simulink library "CTRL_LO_ST3"  (R2023b)
settings: Solver=VariableStepAuto  StartTime=0.0  StopTime=10.0  RelTol=1e-3
undefined symbols (not defined in the file or in its folder): CTRL_LO_p_TqMotLoLim_Nm, CTRL_LO_p_TqMotUpLim_Nm, CTRL_LO_ST3_p_SwtTqFrReRat_na, CTRL_LO_ST3_p_SwtTqYawFrReRat_na, CTRL_LO_ST3_p_TqFrReRat1_na, CTRL_LO_ST3_p_TqFrReRat2_na, CTRL_LO_ST3_p_TqFrReRat3_na, CTRL_LO_ST3_p_TqYawFrReRat1_na, CTRL_LO_ST3_p_TqYawFrReRat2_na, CTRL_LO_ST3_p_TqYawFrReRat3_na, p_RadWhlDynFr_m, p_RadWhlDynRe_m, p_RatGearFr_na, p_trackFr_m, p_trackRe_m
libraries: simulink x1
settings Model: Creator=blatak  LastModifiedBy=blatak

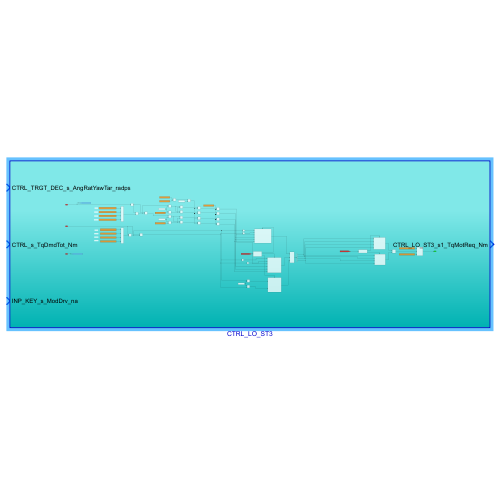
[thumbnail: Simulink's stored preview of the top-level diagram]
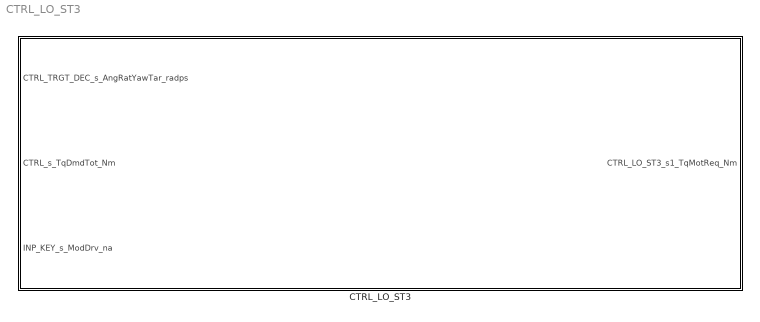
== system CTRL_LO_ST3 ==
  CTRL_LO_ST3 : Subsystem

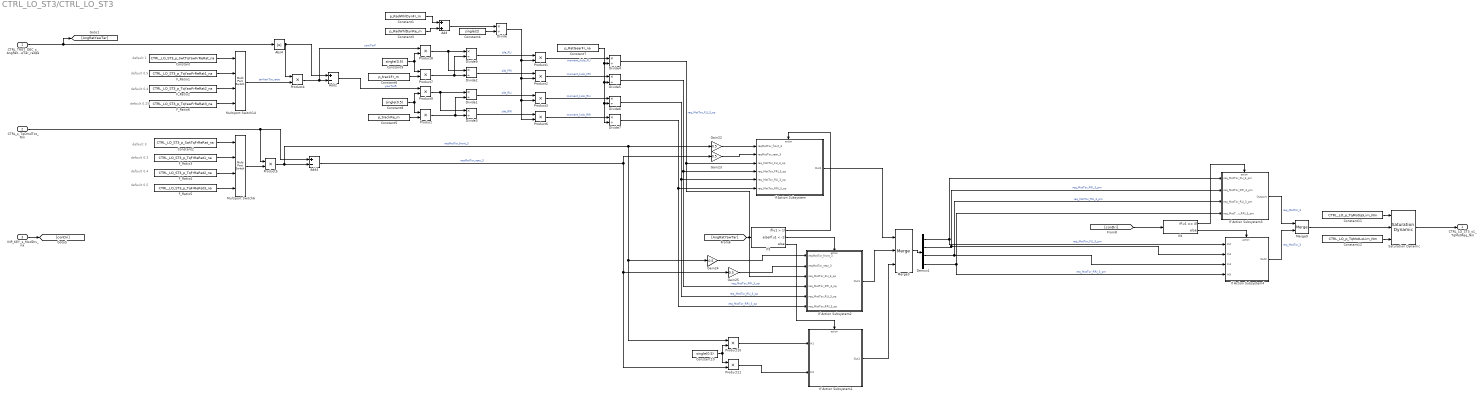
== system CTRL_LO_ST3/CTRL_LO_ST3 ==
  note: default 1
  note: default 0.5
  note: default 0.4
  note: default 0.25
  note: default 0.4
  note: default 0.5
  note: default 3
  note: default 0.3
  CTRL_TRGT_DEC_s_AngRatYawTar_radps : Inport
  CTRL_s_TqDmdTot_Nm : Inport  Port=2
  INP_KEY_s_ModDrv_na : Inport  Port=3
  Abs4 : Abs  SaturateOnIntegerOverflow=off
  Add : Sum
  Add2 : Sum  Inputs=+-
  Add4 : Sum  Inputs=+-
  Constant : Constant  Value=CTRL_LO_ST3_p_SwtTqYawFrReRat_na
  Constant1 : Constant  Value=p_RadWhlDynFr_m
  Constant10 : Constant  Value=single(0.5)
  Constant11 : Constant  Value=CTRL_LO_p_TqMotUpLim_Nm
  Constant12 : Constant  Value=CTRL_LO_p_TqMotLoLim_Nm
  Constant2 : Constant  Value=CTRL_LO_ST3_p_SwtTqFrReRat_na
  Constant3 : Constant  Value=p_RadWhlDynRe_m
  Constant4 : Constant  Value=single(2)
  Constant5 : Constant  Value=p_trackRe_m
  Constant6 : Constant  Value=p_trackFr_m
  Constant7 : Constant  Value=p_RatGearFr_na
  Constant8 : Constant  Value=single(0.5)
  Constant9 : Constant  Value=single(0.5)
  Demux1 : Demux
  Divide{,1..7,9} (9 alike) : Product  Inputs=*/
  F_Ratio1 : Constant  Value=CTRL_LO_ST3_p_TqYawFrReRat1_na
  F_Ratio2 : Constant  Value=CTRL_LO_ST3_p_TqYawFrReRat2_na
  F_Ratio3 : Constant  Value=CTRL_LO_ST3_p_TqFrReRat1_na
  F_Ratio4 : Constant  Value=CTRL_LO_ST3_p_TqFrReRat2_na
  F_Ratio5 : Constant  Value=CTRL_LO_ST3_p_TqFrReRat3_na
  F_Ratio6 : Constant  Value=CTRL_LO_ST3_p_TqYawFrReRat3_na
  Gain{22..25} (4 alike) : Gain  Gain=0.5
  If Action Subsystem : Subsystem  TreatAsAtomicUnit=on
  If Action Subsystem1 : Subsystem  TreatAsAtomicUnit=on
  If Action Subsystem2 : Subsystem  TreatAsAtomicUnit=on
  If Action Subsystem3 : Subsystem  TreatAsAtomicUnit=on
  If Action Subsystem4 : Subsystem  TreatAsAtomicUnit=on
  If3 : If  IfExpression=u1 > 1  ElseIfExpressions=u1 < -1
  If4 : If  IfExpression=u1 == 4
  Merge3 : Merge  Inputs=3
  Merge9 : Merge
  Multiport Switch14 : MultiPortSwitch  SaturateOnIntegerOverflow=off  InputSameDT=off
  Multiport Switch6 : MultiPortSwitch  SaturateOnIntegerOverflow=off  InputSameDT=off
  Product{,1..11} (12 alike) : Product
  Saturation Dynamic : simulink/Discontinuities/Saturation Dynamic  OutMin=[]  OutMax=[]  OutDataTypeStr=Inherit: Same as second input  OutDataType=fixdt(1, 16)  OutScaling=2^-10  DoSatur=off
  CTRL_LO_ST3_s1_TqMotReq_Nm : Outport
  wires:
  If3/2 -> If Action Subsystem2/Action
  Demux1/2 -> If Action Subsystem4/2(In3), If Action Subsystem3/2(req_MotTor_FRI_3_pm)  "req_MotTor_FRI_3_pm"
  If3/1 -> If Action Subsystem/Action
  Product5/1 -> Product10/1, Gain24/1, Gain22/1, Add4/2  "reqMotTor_front_3"
  CTRL_TRGT_DEC_s_AngRatYawTar_radps/1 -> [AngRatYawTar], Abs4/1
  Demux1/3 -> If Action Subsystem4/3(In4), If Action Subsystem3/3(req_MotTor_RLI_3_pm)  "req_MotTor_RLI_3_pm"
  If Action Subsystem/1(Out1) -> Merge3/1
  Demux1/1 -> If Action Subsystem4/1(In2), If Action Subsystem3/1(req_MotTor_FLI_3_pm)  "req_MotTor_FLI_3_pm"
  Divide5/1 -> If Action Subsystem2/4(req_MotTor_FRI_3_op), If Action Subsystem/4(req_MotTor_FRI_3_op)  "req_MotTor_FRI_3_op"
  Product4/1 -> Product8/1, Add2/2  "yawTorF"
  F_Ratio1/1 -> Multiport Switch14/2
  F_Ratio6/1 -> Multiport Switch14/4
  Gain23/1 -> If Action Subsystem/2(reqMotTor_rear_3)
  Divide6/1 -> If Action Subsystem2/5(req_MotTor_RLI_3_op), If Action Subsystem/5(req_MotTor_RLI_3_op)  "req_MotTor_RLI_3_op"
  Add2/1 -> Product9/1  "yawTorR"
  If4/2 -> If Action Subsystem4/Action
  If Action Subsystem4/1(Out2) -> Merge9/2  "req_MotTor_3"
  F_Ratio2/1 -> Multiport Switch14/3
  CTRL_s_TqDmdTot_Nm/1 -> Add4/1, Product5/1
  Abs4/1 -> Add2/1, Product4/1
  Multiport Switch14/1 -> Product4/2  "tarYawTor_ratio"
  Constant2/1 -> Multiport Switch6/1
  F_Ratio3/1 -> Multiport Switch6/2
  Divide4/1 -> If Action Subsystem2/3(req_MotTor_FLI_3_op), If Action Subsystem/3(req_MotTor_FLI_3_op)  "req_MotTor_FLI_3_op"
  Product11/1 -> If Action Subsystem1/2(In2)
  F_Ratio5/1 -> Multiport Switch6/4
  Multiport Switch6/1 -> Product5/2
  Product10/1 -> If Action Subsystem1/1(In1)
  If4/1 -> If Action Subsystem3/Action
  If Action Subsystem2/1(Out1) -> Merge3/2
  F_Ratio4/1 -> Multiport Switch6/3
  [AngRatYawTar] -> If3/1
  If Action Subsystem3/1(Outport) -> Merge9/1  "req_MotTor_3"
  If3/3 -> If Action Subsystem1/Action
  Divide7/1 -> If Action Subsystem2/6(req_MotTor_RRI_3_op), If Action Subsystem/6(req_MotTor_RRI_3_op)  "req_MotTor_RRI_3_op"
  Merge3/1 -> Demux1/1
  Add4/1 -> Product11/2, Gain25/1, Gain23/1  "reqMotTor_rear_3"
  Gain22/1 -> If Action Subsystem/1(reqMotTor_front_3)
  [conDri] -> If4/1
  Gain25/1 -> If Action Subsystem2/2(reqMotTor_rear_3)
  Gain24/1 -> If Action Subsystem2/1(reqMotTor_front_3)
  Constant/1 -> Multiport Switch14/1
  Demux1/4 -> If Action Subsystem3/4(req_MotTor_RRI_3_pm), If Action Subsystem4/4(In5)  "req_MotTor_RRI_3_pm"
  If Action Subsystem1/1(Out1) -> Merge3/3
  Constant6/1 -> Product7/2
  Product2/1 -> Divide5/1  "moment_kolo_FRI"
  Product7/1 -> Divide2/2, Divide9/2
  Product1/1 -> Divide4/1  "moment_kolo_FLI"
  Divide/1 -> Product6/2, Product3/2, Product2/2, Product1/2
  Product/1 -> Divide3/2, Divide1/2
  Divide3/1 -> Product6/1  "sila_RRI"
  Constant5/1 -> Product/2
  Divide1/1 -> Product3/1  "sila_RLI"
  Product6/1 -> Divide7/1  "moment_kolo_RRI"
  Divide9/1 -> Product1/1  "sila_FLI"
  Product8/1 -> Divide9/1, Divide2/1
  Constant7/1 -> Divide4/2, Divide7/2, Divide6/2, Divide5/2
  Divide2/1 -> Product2/1  "sila_FRI"
  Product3/1 -> Divide6/1  "moment_kolo_RLI"
  Product9/1 -> Divide1/1, Divide3/1
  Constant4/1 -> Divide/2
  Add/1 -> Divide/1
  Constant1/1 -> Add/1
  Constant3/1 -> Add/2
  Constant8/1 -> Product9/2, Product/1
  Constant9/1 -> Product7/1, Product8/2
  INP_KEY_s_ModDrv_na/1 -> [conDri]
  Constant10/1 -> Product11/1, Product10/2
  Merge9/1 -> Saturation Dynamic/2
  Constant12/1 -> Saturation Dynamic/3
  Constant11/1 -> Saturation Dynamic/1
  Saturation Dynamic/1 -> CTRL_LO_ST3_s1_TqMotReq_Nm/1

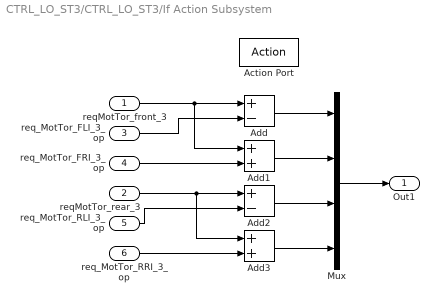
== system CTRL_LO_ST3/CTRL_LO_ST3/If Action Subsystem ==
  reqMotTor_front_3 : Inport
  reqMotTor_rear_3 : Inport  Port=2
  req_MotTor_FLI_3_op : Inport  Port=3
  req_MotTor_FRI_3_op : Inport  Port=4
  req_MotTor_RLI_3_op : Inport  Port=5
  req_MotTor_RRI_3_op : Inport  Port=6
  Action Port : ActionPort  ActionPortLabel=if(u1 > 1)
  Add : Sum  Inputs=+-
  Add1 : Sum
  Add2 : Sum  Inputs=+-
  Add3 : Sum
  Mux : Mux
  Out1 : Outport
  wires:
  req_MotTor_FRI_3_op/1 -> Add1/2
  reqMotTor_front_3/1 -> Add1/1, Add/1
  Add1/1 -> Mux/2
  Add2/1 -> Mux/3
  req_MotTor_RRI_3_op/1 -> Add3/2
  reqMotTor_rear_3/1 -> Add3/1, Add2/1
  Mux/1 -> Out1/1
  req_MotTor_FLI_3_op/1 -> Add/2
  Add3/1 -> Mux/4
  req_MotTor_RLI_3_op/1 -> Add2/2
  Add/1 -> Mux/1

== system CTRL_LO_ST3/CTRL_LO_ST3/If Action Subsystem1 ==
  In1 : Inport
  In2 : Inport  Port=2
  Action Port : ActionPort  ActionPortLabel=else
  Mux : Mux
  Out1 : Outport
  wires:
  In2/1 -> Mux/4, Mux/3
  In1/1 -> Mux/2, Mux/1
  Mux/1 -> Out1/1

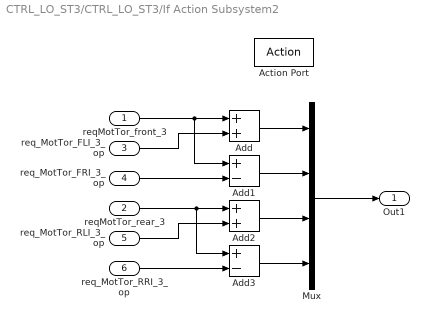
== system CTRL_LO_ST3/CTRL_LO_ST3/If Action Subsystem2 ==
  reqMotTor_front_3 : Inport
  reqMotTor_rear_3 : Inport  Port=2
  req_MotTor_FLI_3_op : Inport  Port=3
  req_MotTor_FRI_3_op : Inport  Port=4
  req_MotTor_RLI_3_op : Inport  Port=5
  req_MotTor_RRI_3_op : Inport  Port=6
  Action Port : ActionPort  ActionPortLabel=elseif(u1 < -1)
  Add : Sum
  Add1 : Sum  Inputs=+-
  Add2 : Sum
  Add3 : Sum  Inputs=+-
  Mux : Mux
  Out1 : Outport
  wires:
  reqMotTor_rear_3/1 -> Add3/1, Add2/1
  req_MotTor_RLI_3_op/1 -> Add2/2
  Mux/1 -> Out1/1
  Add/1 -> Mux/1
  req_MotTor_RRI_3_op/1 -> Add3/2
  req_MotTor_FLI_3_op/1 -> Add/2
  Add2/1 -> Mux/3
  reqMotTor_front_3/1 -> Add1/1, Add/1
  Add1/1 -> Mux/2
  Add3/1 -> Mux/4
  req_MotTor_FRI_3_op/1 -> Add1/2

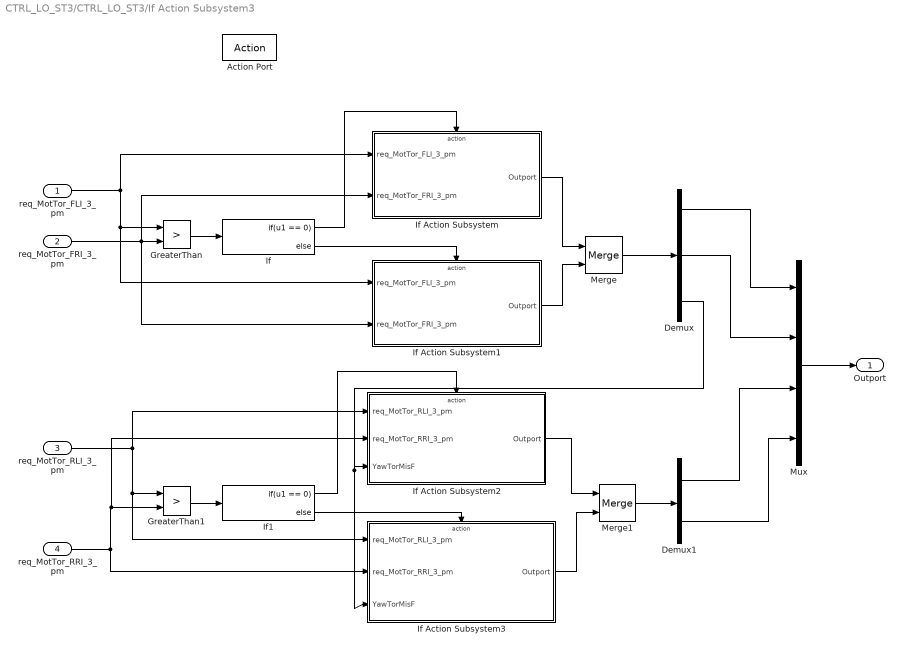
== system CTRL_LO_ST3/CTRL_LO_ST3/If Action Subsystem3 ==
  req_MotTor_FLI_3_pm : Inport
  req_MotTor_FRI_3_pm : Inport  Port=2
  req_MotTor_RLI_3_pm : Inport  Port=3
  req_MotTor_RRI_3_pm : Inport  Port=4
  Action Port : ActionPort  ActionPortLabel=if(u1 == 4)
  Demux : Demux  Outputs=3
  Demux1 : Demux  Outputs=2
  GreaterThan : RelationalOperator  Operator=>  OutDataTypeStr=boolean  RndMeth=Simplest  InputSameDT=off
  GreaterThan1 : RelationalOperator  Operator=>  OutDataTypeStr=boolean  RndMeth=Simplest  InputSameDT=off
  If : If  IfExpression=u1 == 0
  If Action Subsystem : Subsystem  TreatAsAtomicUnit=on
  If Action Subsystem1 : Subsystem  TreatAsAtomicUnit=on
  If Action Subsystem2 : Subsystem  TreatAsAtomicUnit=on
  If Action Subsystem3 : Subsystem  TreatAsAtomicUnit=on
  If1 : If  IfExpression=u1 == 0
  Merge : Merge
  Merge1 : Merge
  Mux : Mux
  Outport : Outport
  wires:
  GreaterThan/1 -> If/1
  If/1 -> If Action Subsystem/Action
  If1/1 -> If Action Subsystem2/Action
  If1/2 -> If Action Subsystem3/Action
  GreaterThan1/1 -> If1/1
  req_MotTor_RLI_3_pm/1 -> If Action Subsystem2/1(req_MotTor_RLI_3_pm), If Action Subsystem3/1(req_MotTor_RLI_3_pm), GreaterThan1/1
  req_MotTor_FRI_3_pm/1 -> If Action Subsystem1/2(req_MotTor_FRI_3_pm), If Action Subsystem/2(req_MotTor_FRI_3_pm), GreaterThan/2
  req_MotTor_RRI_3_pm/1 -> If Action Subsystem3/2(req_MotTor_RRI_3_pm), If Action Subsystem2/2(req_MotTor_RRI_3_pm), GreaterThan1/2
  If/2 -> If Action Subsystem1/Action
  req_MotTor_FLI_3_pm/1 -> If Action Subsystem/1(req_MotTor_FLI_3_pm), If Action Subsystem1/1(req_MotTor_FLI_3_pm), GreaterThan/1
  If Action Subsystem/1(Outport) -> Merge/1
  If Action Subsystem1/1(Outport) -> Merge/2
  If Action Subsystem2/1(Outport) -> Merge1/1
  If Action Subsystem3/1(Outport) -> Merge1/2
  Merge/1 -> Demux/1
  Demux/3 -> If Action Subsystem3/3(YawTorMisF), If Action Subsystem2/3(YawTorMisF)
  Merge1/1 -> Demux1/1
  Demux/1 -> Mux/1
  Demux/2 -> Mux/2
  Demux1/1 -> Mux/3
  Demux1/2 -> Mux/4
  Mux/1 -> Outport/1

== system CTRL_LO_ST3/CTRL_LO_ST3/If Action Subsystem4 ==
  In2 : Inport
  In3 : Inport  Port=2
  In4 : Inport  Port=3
  In5 : Inport  Port=4
  Action Port : ActionPort  ActionPortLabel=else
  Mux : Mux
  Out2 : Outport
  wires:
  Mux/1 -> Out2/1
  In5/1 -> Mux/4
  In3/1 -> Mux/2
  In4/1 -> Mux/3
  In2/1 -> Mux/1

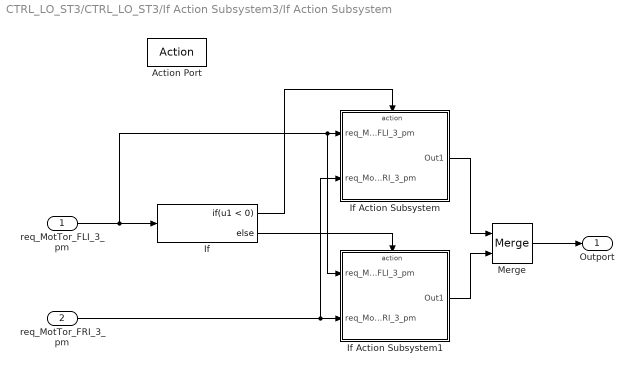
== system CTRL_LO_ST3/CTRL_LO_ST3/If Action Subsystem3/If Action Subsystem ==
  req_MotTor_FLI_3_pm : Inport
  req_MotTor_FRI_3_pm : Inport  Port=2
  Action Port : ActionPort  ActionPortLabel=if(u1 == 0)
  If : If  IfExpression=u1 < 0
  If Action Subsystem : Subsystem  TreatAsAtomicUnit=on
  If Action Subsystem1 : Subsystem  TreatAsAtomicUnit=on
  Merge : Merge
  Outport : Outport
  wires:
  If/1 -> If Action Subsystem/Action
  If/2 -> If Action Subsystem1/Action
  req_MotTor_FRI_3_pm/1 -> If Action Subsystem1/2(req_MotTor_FRI_3_pm), If Action Subsystem/2(req_MotTor_FRI_3_pm)
  req_MotTor_FLI_3_pm/1 -> If Action Subsystem1/1(req_MotTor_FLI_3_pm), If Action Subsystem/1(req_MotTor_FLI_3_pm), If/1
  If Action Subsystem/1(Out1) -> Merge/1
  If Action Subsystem1/1(Out1) -> Merge/2
  Merge/1 -> Outport/1

== system CTRL_LO_ST3/CTRL_LO_ST3/If Action Subsystem3/If Action Subsystem1 ==
  req_MotTor_FLI_3_pm : Inport
  req_MotTor_FRI_3_pm : Inport  Port=2
  Action Port : ActionPort  ActionPortLabel=else
  If : If  IfExpression=u1 < 0
  If Action Subsystem : Subsystem  TreatAsAtomicUnit=on
  If Action Subsystem1 : Subsystem  TreatAsAtomicUnit=on
  Merge : Merge
  Outport : Outport
  wires:
  If/1 -> If Action Subsystem/Action
  If/2 -> If Action Subsystem1/Action
  req_MotTor_FRI_3_pm/1 -> If Action Subsystem1/2(req_MotTor_FRI_3_pm), If Action Subsystem/2(req_MotTor_FRI_3_pm), If/1
  req_MotTor_FLI_3_pm/1 -> If Action Subsystem1/1(req_MotTor_FLI_3_pm), If Action Subsystem/1(req_MotTor_FLI_3_pm)
  If Action Subsystem/1(Out1) -> Merge/1
  If Action Subsystem1/1(Out1) -> Merge/2
  Merge/1 -> Outport/1

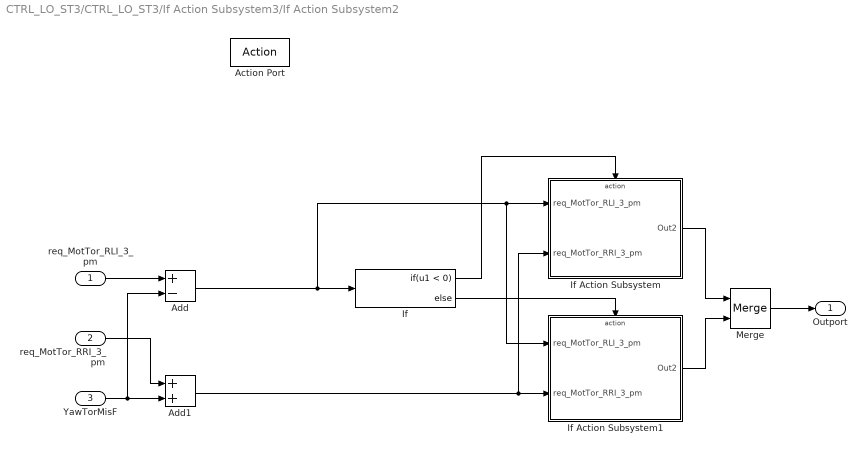
== system CTRL_LO_ST3/CTRL_LO_ST3/If Action Subsystem3/If Action Subsystem2 ==
  req_MotTor_RLI_3_pm : Inport
  req_MotTor_RRI_3_pm : Inport  Port=2
  YawTorMisF : Inport  Port=3
  Action Port : ActionPort  ActionPortLabel=if(u1 == 0)
  Add : Sum  Inputs=+-
  Add1 : Sum
  If : If  IfExpression=u1 < 0
  If Action Subsystem : Subsystem  TreatAsAtomicUnit=on
  If Action Subsystem1 : Subsystem  TreatAsAtomicUnit=on
  Merge : Merge
  Outport : Outport
  wires:
  Add/1 -> If/1, If Action Subsystem1/1(req_MotTor_RLI_3_pm), If Action Subsystem/1(req_MotTor_RLI_3_pm)
  If/1 -> If Action Subsystem/Action
  Add1/1 -> If Action Subsystem1/2(req_MotTor_RRI_3_pm), If Action Subsystem/2(req_MotTor_RRI_3_pm)
  If/2 -> If Action Subsystem1/Action
  req_MotTor_RRI_3_pm/1 -> Add1/1
  req_MotTor_RLI_3_pm/1 -> Add/1
  YawTorMisF/1 -> Add1/2, Add/2
  If Action Subsystem/1(Out2) -> Merge/1
  If Action Subsystem1/1(Out2) -> Merge/2
  Merge/1 -> Outport/1

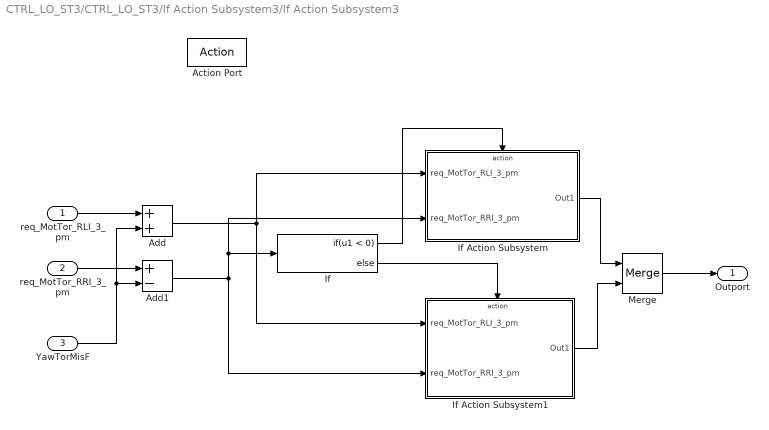
== system CTRL_LO_ST3/CTRL_LO_ST3/If Action Subsystem3/If Action Subsystem3 ==
  req_MotTor_RLI_3_pm : Inport
  req_MotTor_RRI_3_pm : Inport  Port=2
  YawTorMisF : Inport  Port=3
  Action Port : ActionPort  ActionPortLabel=else
  Add : Sum
  Add1 : Sum  Inputs=+-
  If : If  IfExpression=u1 < 0
  If Action Subsystem : Subsystem  TreatAsAtomicUnit=on
  If Action Subsystem1 : Subsystem  TreatAsAtomicUnit=on
  Merge : Merge
  Outport : Outport
  wires:
  req_MotTor_RLI_3_pm/1 -> Add/1
  Add/1 -> If Action Subsystem1/1(req_MotTor_RLI_3_pm), If Action Subsystem/1(req_MotTor_RLI_3_pm)
  req_MotTor_RRI_3_pm/1 -> Add1/1
  If/2 -> If Action Subsystem1/Action
  Add1/1 -> If Action Subsystem1/2(req_MotTor_RRI_3_pm), If Action Subsystem/2(req_MotTor_RRI_3_pm), If/1
  If/1 -> If Action Subsystem/Action
  YawTorMisF/1 -> Add/2, Add1/2
  If Action Subsystem/1(Out1) -> Merge/1
  If Action Subsystem1/1(Out1) -> Merge/2
  Merge/1 -> Outport/1

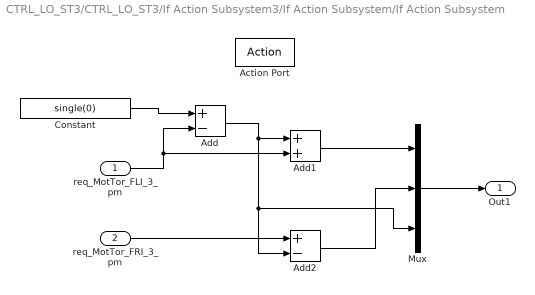
== system CTRL_LO_ST3/CTRL_LO_ST3/If Action Subsystem3/If Action Subsystem/If Action Subsystem ==
  req_MotTor_FLI_3_pm : Inport
  req_MotTor_FRI_3_pm : Inport  Port=2
  Action Port : ActionPort  ActionPortLabel=if(u1 < 0)
  Add : Sum  Inputs=+-
  Add1 : Sum
  Add2 : Sum  Inputs=+-
  Constant : Constant  Value=single(0)
  Mux : Mux  Inputs=3
  Out1 : Outport
  wires:
  Add1/1 -> Mux/1
  Add/1 -> Add2/2, Mux/3, Add1/1
  Add2/1 -> Mux/2
  Constant/1 -> Add/1
  Mux/1 -> Out1/1
  req_MotTor_FRI_3_pm/1 -> Add2/1
  req_MotTor_FLI_3_pm/1 -> Add1/2, Add/2

== system CTRL_LO_ST3/CTRL_LO_ST3/If Action Subsystem3/If Action Subsystem/If Action Subsystem1 ==
  req_MotTor_FLI_3_pm : Inport
  req_MotTor_FRI_3_pm : Inport  Port=2
  Action Port : ActionPort  ActionPortLabel=else
  Constant : Constant  Value=single(0)
  Mux : Mux  Inputs=3
  Out1 : Outport
  wires:
  Mux/1 -> Out1/1
  req_MotTor_FRI_3_pm/1 -> Mux/2
  req_MotTor_FLI_3_pm/1 -> Mux/1
  Constant/1 -> Mux/3

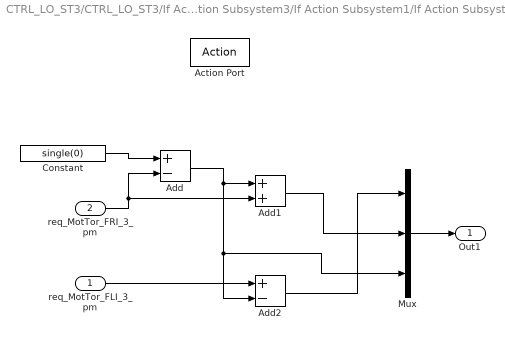
== system CTRL_LO_ST3/CTRL_LO_ST3/If Action Subsystem3/If Action Subsystem1/If Action Subsystem ==
  req_MotTor_FLI_3_pm : Inport
  req_MotTor_FRI_3_pm : Inport  Port=2
  Action Port : ActionPort  ActionPortLabel=if(u1 < 0)
  Add : Sum  Inputs=+-
  Add1 : Sum
  Add2 : Sum  Inputs=+-
  Constant : Constant  Value=single(0)
  Mux : Mux  Inputs=3
  Out1 : Outport
  wires:
  req_MotTor_FLI_3_pm/1 -> Add2/1
  Add/1 -> Add2/2, Mux/3, Add1/1
  Mux/1 -> Out1/1
  Add2/1 -> Mux/1
  Add1/1 -> Mux/2
  req_MotTor_FRI_3_pm/1 -> Add1/2, Add/2
  Constant/1 -> Add/1

== system CTRL_LO_ST3/CTRL_LO_ST3/If Action Subsystem3/If Action Subsystem1/If Action Subsystem1 ==
  req_MotTor_FLI_3_pm : Inport
  req_MotTor_FRI_3_pm : Inport  Port=2
  Action Port : ActionPort  ActionPortLabel=else
  Constant : Constant  Value=single(0)
  Mux : Mux  Inputs=3
  Out1 : Outport
  wires:
  Mux/1 -> Out1/1
  req_MotTor_FLI_3_pm/1 -> Mux/1
  Constant/1 -> Mux/3
  req_MotTor_FRI_3_pm/1 -> Mux/2

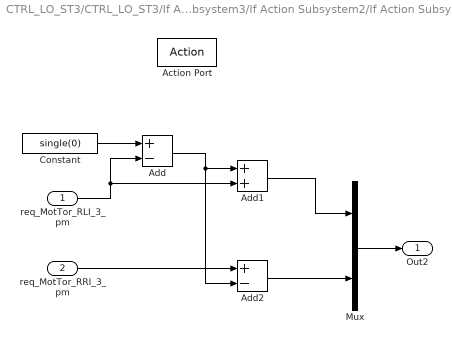
== system CTRL_LO_ST3/CTRL_LO_ST3/If Action Subsystem3/If Action Subsystem2/If Action Subsystem ==
  req_MotTor_RLI_3_pm : Inport
  req_MotTor_RRI_3_pm : Inport  Port=2
  Action Port : ActionPort  ActionPortLabel=if(u1 < 0)
  Add : Sum  Inputs=+-
  Add1 : Sum
  Add2 : Sum  Inputs=+-
  Constant : Constant  Value=single(0)
  Mux : Mux  Inputs=2
  Out2 : Outport
  wires:
  Mux/1 -> Out2/1
  req_MotTor_RRI_3_pm/1 -> Add2/1
  req_MotTor_RLI_3_pm/1 -> Add1/2, Add/2
  Add/1 -> Add2/2, Add1/1
  Constant/1 -> Add/1
  Add1/1 -> Mux/1
  Add2/1 -> Mux/2

== system CTRL_LO_ST3/CTRL_LO_ST3/If Action Subsystem3/If Action Subsystem2/If Action Subsystem1 ==
  req_MotTor_RLI_3_pm : Inport
  req_MotTor_RRI_3_pm : Inport  Port=2
  Action Port : ActionPort  ActionPortLabel=else
  Mux : Mux  Inputs=2
  Out2 : Outport
  wires:
  req_MotTor_RRI_3_pm/1 -> Mux/2
  req_MotTor_RLI_3_pm/1 -> Mux/1
  Mux/1 -> Out2/1

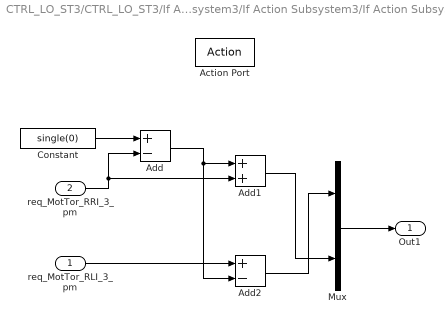
== system CTRL_LO_ST3/CTRL_LO_ST3/If Action Subsystem3/If Action Subsystem3/If Action Subsystem ==
  req_MotTor_RLI_3_pm : Inport
  req_MotTor_RRI_3_pm : Inport  Port=2
  Action Port : ActionPort  ActionPortLabel=if(u1 < 0)
  Add : Sum  Inputs=+-
  Add1 : Sum
  Add2 : Sum  Inputs=+-
  Constant : Constant  Value=single(0)
  Mux : Mux  Inputs=2
  Out1 : Outport
  wires:
  req_MotTor_RLI_3_pm/1 -> Add2/1
  Constant/1 -> Add/1
  Add2/1 -> Mux/1
  Mux/1 -> Out1/1
  Add1/1 -> Mux/2
  req_MotTor_RRI_3_pm/1 -> Add1/2, Add/2
  Add/1 -> Add2/2, Add1/1

== system CTRL_LO_ST3/CTRL_LO_ST3/If Action Subsystem3/If Action Subsystem3/If Action Subsystem1 ==
  req_MotTor_RLI_3_pm : Inport
  req_MotTor_RRI_3_pm : Inport  Port=2
  Action Port : ActionPort  ActionPortLabel=else
  Mux : Mux  Inputs=2
  Out1 : Outport
  wires:
  req_MotTor_RRI_3_pm/1 -> Mux/2
  req_MotTor_RLI_3_pm/1 -> Mux/1
  Mux/1 -> Out1/1
